simulink model "PID_discreto_so_motor_old_version_nuevo"  (R2022b)
settings: Solver=ode4  StartTime=0.0  StopTime=10  FixedStep=0.05  RelTol=1e-3
libraries: sldrtlib x1
settings Model: Creator=Diogo  LastModifiedBy=totti
settings OptimizationCC: ReuseModelBlockBuffer=on

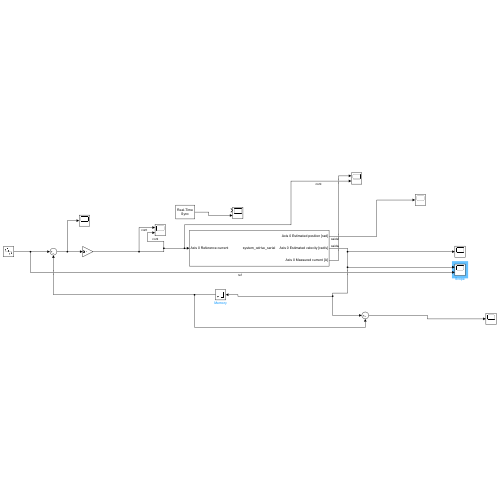
[thumbnail: Simulink's stored preview of the top-level diagram]
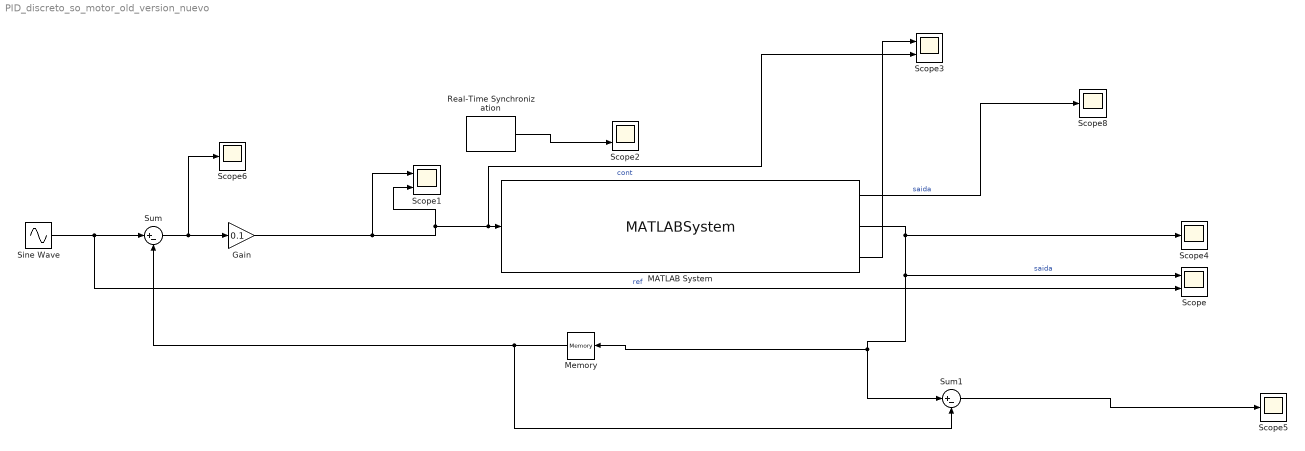
== system PID_discreto_so_motor_old_version_nuevo ==
  Gain : Gain  Gain=0.1
  MATLAB System : MATLABSystem  System=system_odrive_serial  PortName=COM5  Baudrate=115200  Autocalibration=Disabled (fail if not calibrated)  EnableTiming=on  EnableAxis0=on  UseIndex0=off  ResetErrors0=on  ResetPosition0=on  ControlMode0=Position  VelocityLimit0=150  CurrentLimit0=50  TorqueLimit0=1.5  CountsPerRotate0=8192  EnablePosition0Output=on  EnableVelocity0Output=on  EnableCurrent0Output=on  EnableError0Output=off  EnableAxis1=off  CountsPerRotate1=8192  EnablePosition1Output=off  EnableVelocity1Output=off  EnableCurrent1Output=off  EnableError1Output=off  MaxInputParameters=20  Inputs="{  }"  MaxOutputParameters=20  EnableVbusOutput=off  Outputs="{  }"
      mask Type: system_odrive_serial
      mask Display:
      | disp('system_odrive_serial');
      | port_label('input',1,'Axis 0 Reference current');
      | port_label('output',1,'Axis 0 Estimated position [rad]');
      | port_label('output',2,'Axis 0 Estimated velocity [rad/s]');
      | port_label('output',3,'Axis 0 Measured current [A]');
  Memory : Memory
  Real-Time Synchronization : sldrtlib/Real-Time Synchronization  SampleTime=0.05  MaxMissedTicks=1000  ShowMissedTicks=on  YieldWhenWaiting=on
  Scope{,1..3} (4 alike) : Scope  NumInputPorts=2
  Scope{4..6,8} (4 alike) : Scope
  Sine Wave : Sin  Amplitude=10  SampleTime=0
  Sum : Sum  Inputs=|+-
  Sum1 : Sum  Inputs=|+-
  wires:
  Sine Wave/1 -> Scope/2, Sum/1  "ref"
  Sum/1 -> Gain/1, Scope6/1
  MATLAB System/2 -> Memory/1, Sum1/1, Scope/1, Scope4/1  "saida"
  Gain/1 -> Scope3/2, MATLAB System/1, Scope1/2, Scope1/1  "cont"
  Real-Time Synchronization/1 -> Scope2/2
  MATLAB System/3 -> Scope3/1
  MATLAB System/1 -> Scope8/1  "saida"
  Sum1/1 -> Scope5/1
  Memory/1 -> Sum1/2, Sum/2
